simulink model "incre_encoder_new"  (R2020b)
settings: Solver=FixedStepDiscrete  StartTime=0.0  StopTime=0.15  RelTol=1e-3
undefined symbols (not defined in the file): DiscIntNeverNeededParam
libraries: simulink x13, hdlsllib x7
settings Model: DataTypeOverride=Off  Creator=ts  LastModifiedBy=ts
settings DataIOCC: LimitDataPoints=on  SaveOutput=off  SaveTime=off
settings OptimizationCC: BlockReduction=off  ConditionallyExecuteInputs=off  DefaultParameterBehavior=Inlined  LifeSpan=inf
settings DebuggingCC: AlgebraicLoopMsg=error  SingleTaskRateTransMsg=error  AllowSymbolicDim=off  StrictBusMsg=ErrorOnBusTreatedAsVector  SFUnexpectedBacktrackingDiag=warning  SFNoUnconditionalDefaultTransitionDiag=warning  SFExecutionAtInitializationDiag=none  ArithmeticOperatorsInVariantConditions=warning
settings HardwareCC: ProdBitPerPointer=32  ProdBitPerSizeT=32  ProdBitPerPtrDiffT=32  ProdLargestAtomicFloat=None  ProdIntDivRoundTo=Undefined  ProdEndianess=Unspecified  ProdWordSize=32  ProdHWDeviceType=ASIC/FPGA->ASIC/FPGA  ProdEqTarget=off
settings SFSimCC: SimUseLocalCustomCode=off  CustomCodeUndefinedFunction=UseInterfaceOnly
settings RTWCC: RTWUseLocalCustomCode=off
settings CodeAppCC: StateflowObjectComments=on
settings GRTTargetCC: TargetLangStandard=C89/C90 (ANSI)
settings ConfigComp: CovScope=ReferencedModels  CovMetricSettings=dw  CovSaveCumulativeToWorkspaceVar=on  CovSaveSingleToWorkspaceVar=on  CovExternalEMLEnable=off  CovSFcnEnable=off

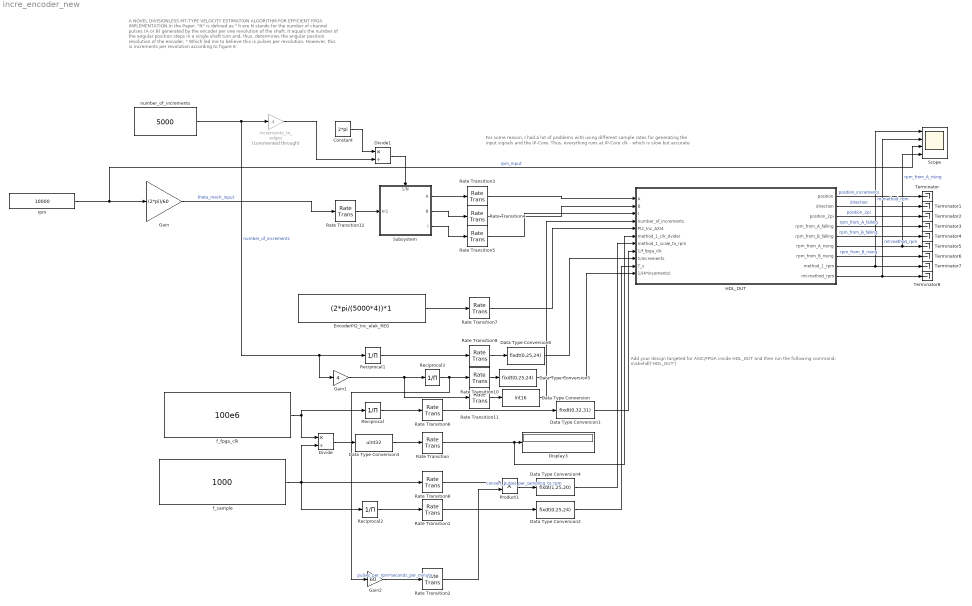
== system incre_encoder_new ==
  note: A NOVEL DIVISIONLESS MT-TYPE VELOCITY
      | ESTIMATION ALGORITHM FOR EFFICIENT
      | FPGA IMPLEMENTATION
      |
      | In the Paper, "N" is defined as " h ere N stands for the number of channel pulses (A or B) generated by the encoder per one revolution of the shaft. It
      | equals the number of the angular position steps in a single
      | shaft turn and, thus, determines the angular position resolution
      | of the encoder. "
      | Which led me to believe this is pulses per revolution. However, this is increments per revolution according to figure 6
  note: For some reason, I had a lot of problems with using different sample rates for generating the input signals and the IP-Core. Thus, everything runs at IP-Core clk - which is slow but accurate
  note: Add your design targeted for ASIC/FPGA inside HDL_DUT and then run the following command:
      | makehdl('HDL_DUT')
  Constant : Constant  Value=2*pi
  Data Type Conversion : DataTypeConversion  OutDataTypeStr=int16
  Data Type Conversion1 : DataTypeConversion  OutDataTypeStr=fixdt(0,32,31)
  Data Type Conversion2 : DataTypeConversion  OutMin=0  OutMax=0.01  OutDataTypeStr=fixdt(0,25,24)
  Data Type Conversion3 : DataTypeConversion  OutDataTypeStr=uint32
  Data Type Conversion4 : DataTypeConversion  OutDataTypeStr=fixdt(1,25,20)
  Data Type Conversion5 : DataTypeConversion  OutDataTypeStr=fixdt(0,25,24)
  Data Type Conversion6 : DataTypeConversion  OutDataTypeStr=fixdt(0,25,24)
  Display3 : Display
  Divide : Product  Inputs=*/
  Divide1 : Product  Inputs=*/
  EncoderPI2_Inc_elek_REG : Constant  Value=(2*pi/(5000*4))*1  OutDataTypeStr=fixdt(0,24,24)  SampleTime=-1
  Gain : Gain  Gain=(2*pi)/60
  Gain1 : Gain  Gain=4
  Gain2 : Gain  Gain=60
  HDL_DUT : Subsystem  TreatAsAtomicUnit=on
  Product1 : Product
  Rate Transition{,1..2,8,12} (5 alike) : RateTransition
  Rate Transition{3..7,9..11} (8 alike) : RateTransition  OutPortSampleTime=1/100e6
  Reciprocal{,1..3} (4 alike) : Product  Inputs=/
  Scope : Scope  NumInputPorts=4
  Subsystem : Subsystem
      settings: PortSchema="{\"entries\":[{\"content\":{\"sides\":[{\"content\":{\"connectorIds\":[\"In1\"]},\"type\":\"ConnectorPlacement.EquallySpacedRectSide\",\"uuid\":\"9e0d3c7a-ae59-4f05-b933-dde2182720d4\"},{\"content\":{\"connectorIds\":[\"Out1\",\"Out2\",\"Out3\"],\"side\":\"RIGHT\"},\"type\":\"ConnectorPlacement.EquallySpacedRectSide\",\"uuid\":\"061efe66-90e8-497d-a95d-e4bb14f2a7fd\"},{\"content\":{\"connectorIds\":[\"In2\"],\"side\":\"TOP\"},\"type\":\"ConnectorPlacement.EquallySpacedRectSide\",\"uuid\":\"3388cf49-edab-4489-bb14-c96d905dcdcb\"},{\"content\":{\"connectorIds\":[],\"side\":\"HIDDEN\"},\"type\":\"ConnectorPlacement.EquallySpacedRectSide\",\"uuid\":\"d7306302-0393-400a-9a2a-0d99055afcd2\"}]},\"type\":\"ConnectorPlacement.EquallySpacedConnector\",\"uuid\":\"eafc6ed9-e172-404f-862e-caf1c3fcd6e0\"}],\"packageUris\":[\"http://schema.mathworks.com/mf0/Connector/R2020b\"],\"version\":\"1.0\"}"
  Terminator{,1..8} (9 alike) : Terminator
  f_fpga_clk : Constant  Value=100e6
  f_sample : Constant  Value=1000
  increments_to_edges : Gain  Commented=through  Gain=4
  number_of_increments : Constant  Value=5000
  rpm : Constant  Value=10000
  wires:
  EncoderPI2_Inc_elek_REG/1 -> Rate Transition7/1
  Rate Transition3/1 -> HDL_DUT/1(A)
  Rate Transition4/1 -> HDL_DUT/2(B)
  Rate Transition5/1 -> HDL_DUT/3(I)
  Data Type Conversion/1 -> HDL_DUT/4(number_of_increments)
  Rate Transition7/1 -> HDL_DUT/5(PI2_Inc_AXI4)
  Product1/1 -> Data Type Conversion4/1  "convert_pulses_per_sampling_to_rpm"
  Rate Transition/1 -> HDL_DUT/6(method_1_clk_dvider), Display3/1
  Data Type Conversion3/1 -> Rate Transition/1
  f_fpga_clk/1 -> Reciprocal/1, Divide/1
  Divide/1 -> Data Type Conversion3/1
  Rate Transition8/1 -> Product1/1
  Reciprocal3/1 -> Gain2/1, Rate Transition10/1
  f_sample/1 -> Reciprocal2/1, Rate Transition8/1, Divide/2
  Rate Transition2/1 -> Product1/2
  Data Type Conversion4/1 -> HDL_DUT/7(method_1_scale_to_rpm)
  Gain/1 -> Rate Transition12/1  "theta_mech_input"
  number_of_increments/1 -> increments_to_edges/1, Gain1/1, Reciprocal1/1  "number_of_increments"
  Subsystem/1(A) -> Rate Transition3/1
  Subsystem/2(B) -> Rate Transition4/1
  Subsystem/3(I) -> Rate Transition5/1
  Reciprocal/1 -> Rate Transition6/1
  Reciprocal1/1 -> Rate Transition9/1
  Reciprocal2/1 -> Rate Transition1/1
  Rate Transition1/1 -> Data Type Conversion2/1
  HDL_DUT/1(position) -> Terminator/1  "position_increments"
  HDL_DUT/2(direction) -> Terminator1/1  "direction"
  HDL_DUT/3(position_2pi) -> Terminator2/1  "position_2pi"
  HDL_DUT/4(rpm_from_A_falling) -> Terminator3/1  "rpm_from_A_falling"
  HDL_DUT/5(rpm_from_B_falling) -> Terminator4/1  "rpm_from_B_falling"
  HDL_DUT/6(rpm_from_A_rising) -> Scope/4, Terminator5/1  "rpm_from_A_rising"
  HDL_DUT/7(rpm_from_B_rising) -> Terminator6/1  "rpm_from_B_rising"
  HDL_DUT/8(method_1_rpm) -> Scope/1, Terminator7/1  "m-method_rpm"
  HDL_DUT/9(mt-method_rpm) -> Scope/2, Terminator8/1  "mt-method_rpm"
  rpm/1 -> Scope/3, Gain/1  "rpm_input"
  Gain1/1 -> Rate Transition11/1, Reciprocal3/1
  Rate Transition9/1 -> Data Type Conversion6/1
  Rate Transition10/1 -> Data Type Conversion5/1
  Rate Transition11/1 -> Data Type Conversion/1
  Gain2/1 -> Rate Transition2/1  "pulses_per_rpm*seconds_per_minute"
  Rate Transition6/1 -> Data Type Conversion1/1
  Data Type Conversion1/1 -> HDL_DUT/8(1/f_fpga_clk)
  Data Type Conversion2/1 -> HDL_DUT/10(T_s)
  Data Type Conversion5/1 -> HDL_DUT/11(1/(4*incements))
  Data Type Conversion6/1 -> HDL_DUT/9(1/increments)
  Rate Transition12/1 -> Subsystem/1(In1)
  increments_to_edges/1 -> Divide1/2
  Divide1/1 -> Subsystem/2(1/N)
  Constant/1 -> Divide1/1

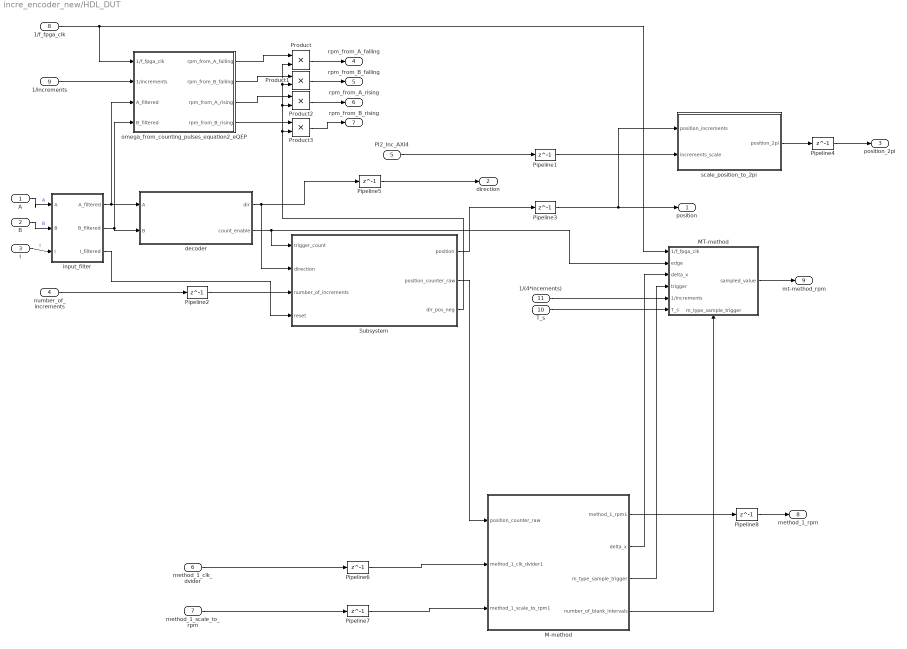
== system incre_encoder_new/HDL_DUT ==
  A : Inport
  B : Inport  Port=2
  I : Inport  Port=3
  number_of_increments : Inport  Port=4
  PI2_Inc_AXI4 : Inport  Port=5
  method_1_clk_dvider : Inport  Port=6
  method_1_scale_to_rpm : Inport  Port=7
  1/f_fpga_clk : Inport  Port=8
  1/increments : Inport  Port=9
  T_s : Inport  Port=10
  1/(4*incements) : Inport  Port=11
  M-method : Subsystem
  MT-method : Subsystem
      settings: PortSchema="{\"entries\":[{\"content\":{\"sides\":[{\"content\":{\"connectorIds\":[\"In1\",\"In2\",\"In3\",\"In4\",\"In5\",\"In6\"]},\"type\":\"ConnectorPlacement.EquallySpacedRectSide\",\"uuid\":\"ebb99f89-30f8-4ce6-b03f-8a2ff0950a3c\"},{\"content\":{\"connectorIds\":[\"Out1\"],\"side\":\"RIGHT\"},\"type\":\"ConnectorPlacement.EquallySpacedRectSide\",\"uuid\":\"75715ffe-4c0f-456c-8ce5-493fcfe41ee3\"},{\"content\":{\"connectorIds\":[],\"side\":\"TOP\"},\"type\":\"ConnectorPlacement.EquallySpacedRectSide\",\"uuid\":\"211c38e6-7e18-4a6c-98ce-7e5618ad5874\"},{\"content\":{\"connectorIds\":[\"In7\"],\"side\":\"BOTTOM\"},\"type\":\"ConnectorPlacement.EquallySpacedRectSide\",\"uuid\":\"87a6a744-1d19-4fed-b30a-33a6e99221e9\"},{\"content\":{\"connectorIds\":[],\"side\":\"HIDDEN\"},\"type\":\"ConnectorPlacement.EquallySpacedRectSide\",\"uuid\":\"5f32e9d6-05c7-4b0a-95ef-6efe95f3ff8d\"}]},\"type\":\"ConnectorPlacement.EquallySpacedConnector\",\"uuid\":\"473bacac-5052-4058-8fec-e1b83cc6224c\"}],\"packageUris\":[\"http://schema.mathworks.com/mf0/Connector/R2020b\"],\"version\":\"1.0\"}"
  Pipeline{1..8} (8 alike) : Delay  DelayLength=1
  Product{,1..3} (4 alike) : Product  OutDataTypeStr=fixdt(1,18,3)
  Subsystem : Subsystem
  decoder : Subsystem
  input_filter : Subsystem
  omega_from_counting_pulses_equation2_eQEP : Subsystem
  scale_position_to_2pi : Subsystem
  position : Outport  VectorParamsAs1DForOutWhenUnconnected=off
  direction : Outport  Port=2
  position_2pi : Outport  Port=3  VectorParamsAs1DForOutWhenUnconnected=off
  rpm_from_A_falling : Outport  Port=4
  rpm_from_B_falling : Outport  Port=5
  rpm_from_A_rising : Outport  Port=6
  rpm_from_B_rising : Outport  Port=7
  method_1_rpm : Outport  Port=8
  mt-method_rpm : Outport  Port=9
  wires:
  Pipeline3/1 -> position/1, scale_position_to_2pi/1(position_increments)
  input_filter/1(A_filtered) -> decoder/1(A), omega_from_counting_pulses_equation2_eQEP/3(A_filtered)
  decoder/1(dir) -> Pipeline5/1, Subsystem/2(direction)
  decoder/2(count_enable) -> Subsystem/1(trigger_count), MT-method/2(edge)
  input_filter/3(I_filtered) -> Subsystem/4(reset)
  Pipeline8/1 -> method_1_rpm/1
  Pipeline4/1 -> position_2pi/1
  Pipeline7/1 -> M-method/3(method_1_scale_to_rpm1)
  Pipeline1/1 -> scale_position_to_2pi/2(increments_scale)
  1/f_fpga_clk/1 -> omega_from_counting_pulses_equation2_eQEP/1(1/f_fpga_clk), MT-method/1(1/f_fpga_clk)
  B/1 -> input_filter/2(B)  "B"
  Pipeline5/1 -> direction/1
  PI2_Inc_AXI4/1 -> Pipeline1/1
  MT-method/1(sampled_value) -> mt-method_rpm/1
  scale_position_to_2pi/1(position_2pi) -> Pipeline4/1
  Subsystem/2(position_counter_raw) -> M-method/1(position_counter_raw)
  T_s/1 -> MT-method/6(T_s)
  A/1 -> input_filter/1(A)  "A"
  method_1_clk_dvider/1 -> Pipeline6/1
  input_filter/2(B_filtered) -> decoder/2(B), omega_from_counting_pulses_equation2_eQEP/4(B_filtered)
  Pipeline2/1 -> Subsystem/3(number_of_increments)
  method_1_scale_to_rpm/1 -> Pipeline7/1
  I/1 -> input_filter/3(I)  "I"
  Subsystem/1(position) -> Pipeline3/1
  Pipeline6/1 -> M-method/2(method_1_clk_dvider1)
  1/increments/1 -> omega_from_counting_pulses_equation2_eQEP/2(1/increments)
  number_of_increments/1 -> Pipeline2/1
  1/(4*incements)/1 -> MT-method/5(1/increments)
  M-method/4(number_of_blank_intervals) -> MT-method/7(m_type_sample_trigger)
  M-method/2(delta_x) -> MT-method/3(delta_x)
  M-method/3(m_type_sample_trigger) -> MT-method/4(trigger)
  M-method/1(method_1_rpm1) -> Pipeline8/1
  Product/1 -> rpm_from_A_falling/1
  Product1/1 -> rpm_from_B_falling/1
  Product2/1 -> rpm_from_A_rising/1
  Product3/1 -> rpm_from_B_rising/1
  Subsystem/3(dir_pos_neg) -> Product3/2, Product2/2, Product1/2, Product/2
  omega_from_counting_pulses_equation2_eQEP/4(rpm_from_B_rising) -> Product3/1
  omega_from_counting_pulses_equation2_eQEP/3(rpm_from_A_rising) -> Product2/1
  omega_from_counting_pulses_equation2_eQEP/2(rpm_from_B_falling) -> Product1/1
  omega_from_counting_pulses_equation2_eQEP/1(rpm_from_A_falling) -> Product/1

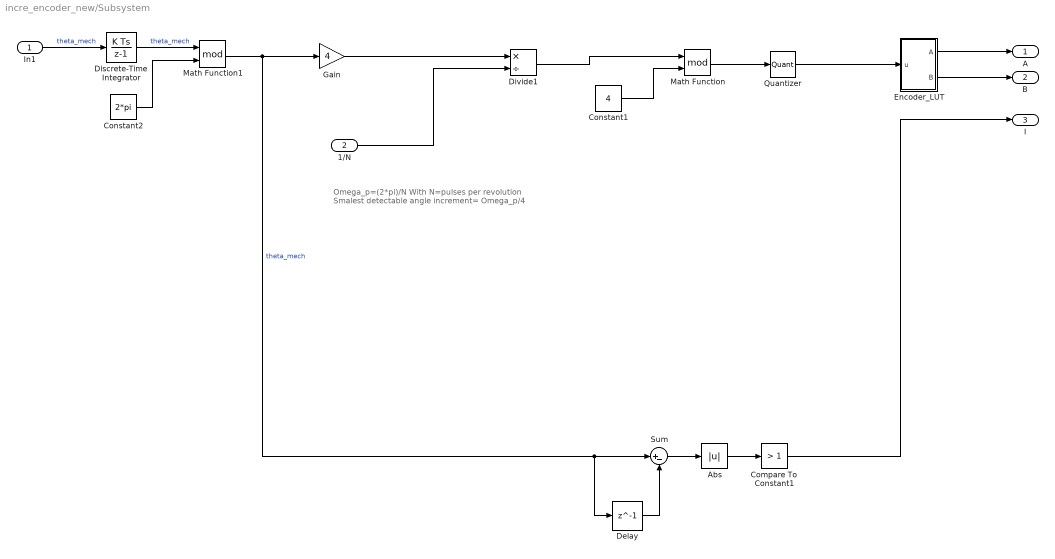
== system incre_encoder_new/Subsystem ==
  note: Omega_p=(2*pi)/N
      | With N=pulses per revolution
      | Smalest detectable angle increment= Omega_p/4
  In1 : Inport
  1/N : Inport  Port=2
  Abs : Abs
  Compare To Constant1 : simulink/Logic and Bit Operations/Compare To Constant  relop=>  const=1  OutDataTypeStr=boolean
  Constant1 : Constant  Value=4
  Constant2 : Constant  Value=2*pi  SampleTime=-1
  Delay : Delay  DelayLength=1
  Discrete-Time Integrator : DiscreteIntegrator  SampleTime=1/100000000  ICPrevOutput=DiscIntNeverNeededParam  ICPrevScaledInput=DiscIntNeverNeededParam
  Divide1 : Product  Inputs=*/
  Encoder_LUT : Subsystem
  Gain : Gain  Gain=4
  Math Function : Math  Operator=mod  SaturateOnIntegerOverflow=on
  Math Function1 : Math  Operator=mod  SaturateOnIntegerOverflow=on
  Quantizer : Quantizer  QuantizationInterval=1
  Sum : Sum  Inputs=|+-
  A : Outport
  B : Outport  Port=2
  I : Outport  Port=3
  wires:
  Gain/1 -> Divide1/1
  Divide1/1 -> Math Function/1
  Constant1/1 -> Math Function/2
  Math Function/1 -> Quantizer/1
  Quantizer/1 -> Encoder_LUT/1(u)
  Encoder_LUT/1(A) -> A/1
  Encoder_LUT/2(B) -> B/1
  Sum/1 -> Abs/1
  Delay/1 -> Sum/2
  Math Function1/1 -> Delay/1, Sum/1, Gain/1  "theta_mech"
  Abs/1 -> Compare To Constant1/1
  Compare To Constant1/1 -> I/1
  Discrete-Time Integrator/1 -> Math Function1/1  "theta_mech"
  Constant2/1 -> Math Function1/2
  In1/1 -> Discrete-Time Integrator/1  "theta_mech"
  1/N/1 -> Divide1/2

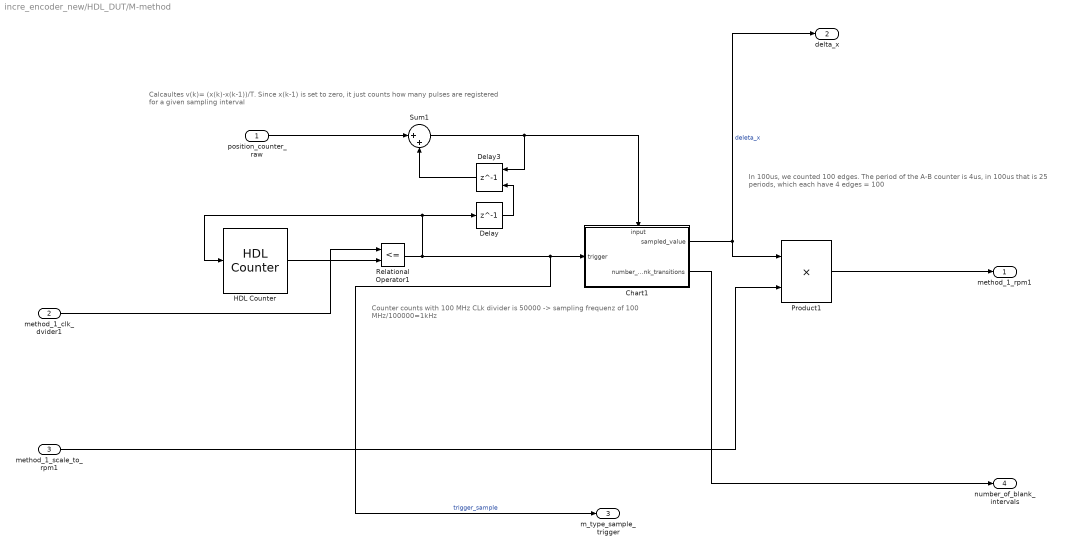
== system incre_encoder_new/HDL_DUT/M-method ==
  note: In 100us, we counted 100 edges.
      | The period of the A-B counter is 4us, in 100us that is 25 periods, which each have 4 edges = 100
  note: Counter counts with 100 MHz
      | CLk divider is 50000 -> sampling frequenz of 100 MHz/100000=1kHz
  note: Calcaultes v(k)= (x(k)-x(k-1))/T. Since x(k-1) is set to zero, it just counts how many pulses are registered for a given sampling interval
  position_counter_raw : Inport
  method_1_clk_dvider1 : Inport  Port=2
  method_1_scale_to_rpm1 : Inport  Port=3
  Chart1 : Stateflow chart  TreatAsAtomicUnit=on
      settings: PortSchema="{\"entries\":[{\"content\":{\"sides\":[{\"content\":{\"connectorIds\":[\"In2\"]},\"type\":\"ConnectorPlacement.EquallySpacedRectSide\",\"uuid\":\"939b8621-78f7-42aa-87b8-407a8b6a498a\"},{\"content\":{\"connectorIds\":[\"Out1\",\"Out2\"],\"side\":\"RIGHT\"},\"type\":\"ConnectorPlacement.EquallySpacedRectSide\",\"uuid\":\"3b067427-2d1d-4835-b293-703ef05eeccb\"},{\"content\":{\"connectorIds\":[\"In1\"],\"side\":\"TOP\"},\"type\":\"ConnectorPlacement.EquallySpacedRectSide\",\"uuid\":\"a3c90177-c936-46a5-9ed2-0ec0dd680635\"},{\"content\":{\"connectorIds\":[],\"side\":\"HIDDEN\"},\"type\":\"ConnectorPlacement.EquallySpacedRectSide\",\"uuid\":\"01f333f2-54e6-42b9-9b27-8dc26f013eb2\"}]},\"type\":\"ConnectorPlacement.EquallySpacedConnector\",\"uuid\":\"7e8a03bf-356f-48c3-b34e-0f0bd6eb938b\"}],\"packageUris\":[\"http://schema.mathworks.com/mf0/Connector/R2020b\"],\"version\":\"1.0\"}"
  Delay : Delay  DelayLength=1
  Delay3 : Delay  DelayLength=1  ExternalReset=Level
      settings: InputPortMap=u0,r5
  HDL Counter : hdlsllib/Sources/HDL Counter  CountType=Free running  CountInit=0  CountStep=1  CountMax=100  CountFromType=Initial value  CountFrom=0  CountResetPort=on  CountLoadPort=off  CountEnbPort=off  CountDirPort=off  CountDataType=Unsigned  CountWordLen=32  CountFracLen=0  CountSampTime=1
  Product1 : Product  OutDataTypeStr=fixdt(1,32,14)
  Relational Operator1 : RelationalOperator  Operator=<=  OutDataTypeStr=boolean  RndMeth=Simplest
  Sum1 : Sum  Inputs=|++  OutDataTypeStr=int32
  method_1_rpm1 : Outport
  delta_x : Outport  Port=2
  m_type_sample_trigger : Outport  Port=3
  number_of_blank_intervals : Outport  Port=4
  wires:
  method_1_scale_to_rpm1/1 -> Product1/2
  Chart1/1(sampled_value) -> Product1/1, delta_x/1  "deleta_x"
  Product1/1 -> method_1_rpm1/1
  position_counter_raw/1 -> Sum1/1
  Delay/1 -> Delay3/2
  Delay3/1 -> Sum1/2
  Sum1/1 -> Delay3/1, Chart1/1(input)
  method_1_clk_dvider1/1 -> Relational Operator1/1
  HDL Counter/1 -> Relational Operator1/2
  Relational Operator1/1 -> Delay/1, HDL Counter/1, m_type_sample_trigger/1, Chart1/2(trigger)  "trigger_sample"
  Chart1/2(number_of_blank_transitions) -> number_of_blank_intervals/1

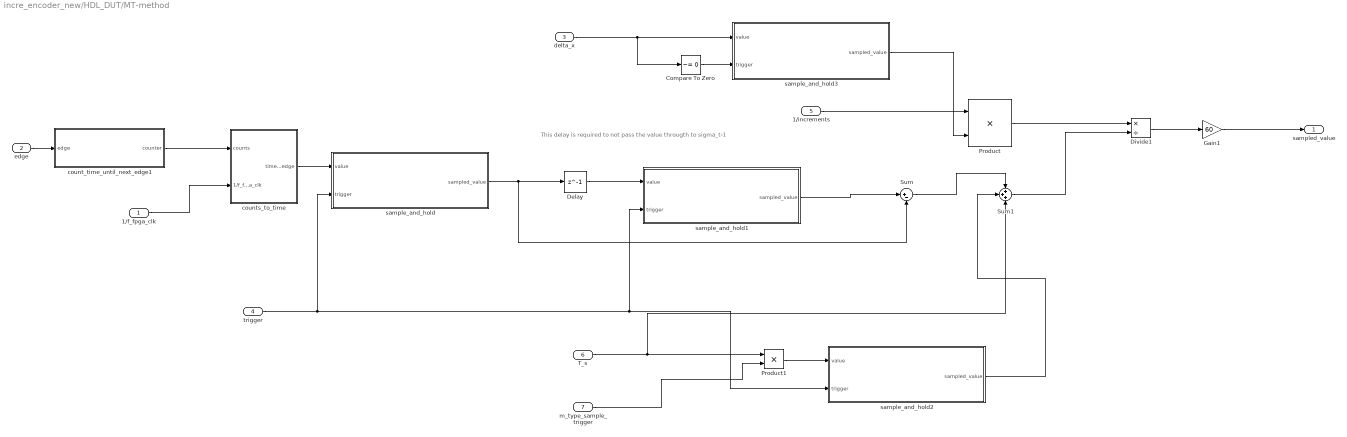
== system incre_encoder_new/HDL_DUT/MT-method ==
  note: This delay is required to not pass the value througth to sigma_t-1
  1/f_fpga_clk : Inport
  edge : Inport  Port=2
  delta_x : Inport  Port=3
  trigger : Inport  Port=4
  1/increments : Inport  Port=5
  T_s : Inport  Port=6
  m_type_sample_trigger : Inport  Port=7
  Compare To Zero : simulink/Logic and Bit Operations/Compare To Zero  relop=~=  OutDataTypeStr=boolean
  Delay : Delay  DelayLength=1
  Divide1 : Product  Inputs=*/  OutDataTypeStr=fixdt(1,18,4)
  Gain1 : Gain  Gain=60  OutDataTypeStr=fixdt(1,18,3)
  Product : Product
  Product1 : Product  OutDataTypeStr=Inherit: Same as first input
  Sum : Sum  Inputs=|+-
  Sum1 : Sum  Inputs=+++
  count_time_until_next_edge1 : Subsystem
  counts_to_time : Subsystem
  sample_and_hold : Subsystem
  sample_and_hold1 : Subsystem
  sample_and_hold2 : Subsystem
  sample_and_hold3 : Subsystem
  sampled_value : Outport
  wires:
  sample_and_hold/1(sampled_value) -> Delay/1, Sum/2
  sample_and_hold1/1(sampled_value) -> Sum/1
  count_time_until_next_edge1/1(counter) -> counts_to_time/1(counts)
  counts_to_time/1(time_since_last_edge) -> sample_and_hold/1(value)
  1/f_fpga_clk/1 -> counts_to_time/2(1/f_fpga_clk)
  delta_x/1 -> Compare To Zero/1, sample_and_hold3/1(value)
  Sum1/1 -> Divide1/2
  sample_and_hold2/1(sampled_value) -> Sum1/2
  Sum/1 -> Sum1/1
  Divide1/1 -> Gain1/1
  edge/1 -> count_time_until_next_edge1/1(edge)
  trigger/1 -> sample_and_hold/2(trigger), sample_and_hold2/2(trigger), sample_and_hold1/2(trigger)
  Delay/1 -> sample_and_hold1/1(value)
  1/increments/1 -> Product/1
  Product/1 -> Divide1/1
  T_s/1 -> Product1/1, Sum1/3
  m_type_sample_trigger/1 -> Product1/2
  Product1/1 -> sample_and_hold2/1(value)
  Compare To Zero/1 -> sample_and_hold3/2(trigger)
  Gain1/1 -> sampled_value/1
  sample_and_hold3/1(sampled_value) -> Product/2

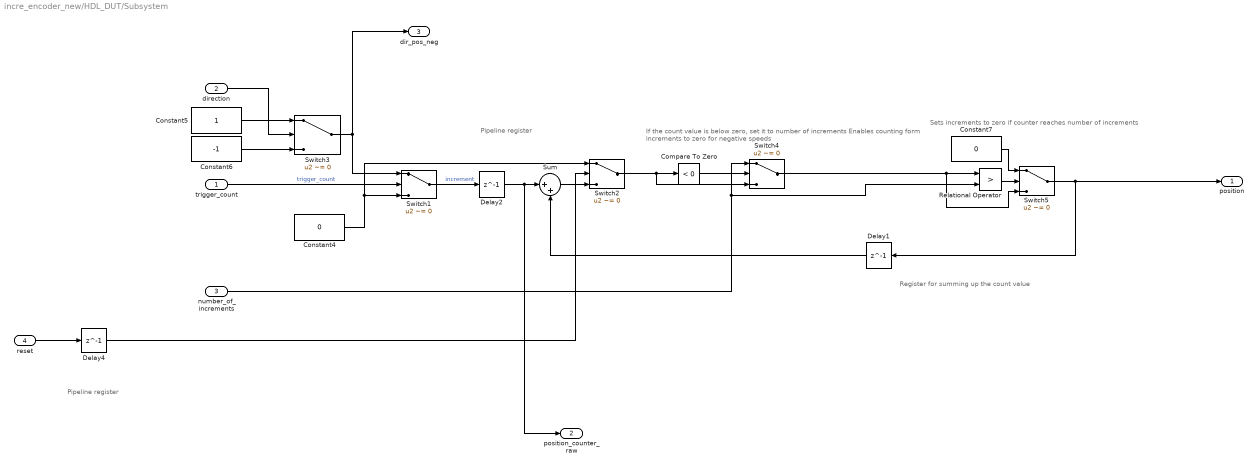
== system incre_encoder_new/HDL_DUT/Subsystem ==
  note: Pipeline register
  note: Register for summing up the count value
  note: Pipeline register
  note: If the count value is below zero, set it to number of increments
      | Enables counting form increments to zero for negative speeds
  note: Sets increments to zero if counter reaches number of increments
  trigger_count : Inport
  direction : Inport  Port=2
  number_of_increments : Inport  Port=3
  reset : Inport  Port=4
  Compare To Zero : simulink/Logic and Bit Operations/Compare To Zero  relop=<  OutDataTypeStr=boolean
  Constant4 : Constant  Value=0  OutDataTypeStr=Inherit: Inherit via back propagation  SampleTime=-1
  Constant5 : Constant  OutDataTypeStr=int16  SampleTime=-1
  Constant6 : Constant  Value=-1  OutDataTypeStr=int16  SampleTime=-1
  Constant7 : Constant  Value=0  OutDataTypeStr=int16  SampleTime=-1
  Delay1 : Delay  DelayLength=1
  Delay2 : Delay  DelayLength=1
  Delay4 : Delay  DelayLength=1
  Relational Operator : RelationalOperator  Operator=>  OutDataTypeStr=boolean  RndMeth=Nearest
  Sum : Sum  Inputs=|++  OutDataTypeStr=int16
  Switch{1..5} (5 alike) : Switch  Criteria=u2 ~= 0
  position : Outport
  position_counter_raw : Outport  Port=2
  dir_pos_neg : Outport  Port=3
  wires:
  Switch3/1 -> Switch1/1, dir_pos_neg/1
  Relational Operator/1 -> Switch5/2
  number_of_increments/1 -> Relational Operator/2, Switch4/1
  trigger_count/1 -> Switch1/2  "trigger_count"
  Constant7/1 -> Switch5/1
  direction/1 -> Switch3/2
  Switch2/1 -> Switch4/3, Compare To Zero/1
  Constant5/1 -> Switch3/1
  Switch5/1 -> position/1, Delay1/1
  Compare To Zero/1 -> Switch4/2
  Constant6/1 -> Switch3/3
  Switch1/1 -> Delay2/1  "increment"
  Delay1/1 -> Sum/2
  Switch4/1 -> Switch5/3, Relational Operator/1
  Constant4/1 -> Switch2/1, Switch1/3
  Sum/1 -> Switch2/3
  reset/1 -> Delay4/1
  Delay2/1 -> position_counter_raw/1, Sum/1
  Delay4/1 -> Switch2/2

== system incre_encoder_new/HDL_DUT/decoder ==
  A : Inport
  B : Inport  Port=2
  Bit Concat : hdlsllib/Logic and Bit Operations/Bit Concat  numInputs=2
  Chart : Stateflow chart  TreatAsAtomicUnit=on
      settings: PortSchema="{\"entries\":[{\"content\":{\"sides\":[{\"content\":{\"connectorIds\":[]},\"type\":\"ConnectorPlacement.EquallySpacedRectSide\",\"uuid\":\"daec34c6-1702-4005-aa49-10d4da34fe8f\"},{\"content\":{\"connectorIds\":[\"Out1\",\"Out2\"],\"side\":\"RIGHT\"},\"type\":\"ConnectorPlacement.EquallySpacedRectSide\",\"uuid\":\"001a9971-efab-40d0-ade0-c56900f25f3e\"},{\"content\":{\"connectorIds\":[\"In1\"],\"side\":\"TOP\"},\"type\":\"ConnectorPlacement.EquallySpacedRectSide\",\"uuid\":\"df9ef995-f205-435f-b234-17c3810a159e\"},{\"content\":{\"connectorIds\":[],\"side\":\"BOTTOM\"},\"type\":\"ConnectorPlacement.EquallySpacedRectSide\",\"uuid\":\"072d0b79-3392-4d8b-8dd8-d2187887a025\"},{\"content\":{\"connectorIds\":[],\"side\":\"HIDDEN\"},\"type\":\"ConnectorPlacement.EquallySpacedRectSide\",\"uuid\":\"c66a1be6-76cb-49b8-a915-e16581d132f1\"}]},\"type\":\"ConnectorPlacement.EquallySpacedConnector\",\"uuid\":\"6a8040ac-5c18-4913-8e6b-fe8fb202e8f4\"}],\"packageUris\":[\"http://schema.mathworks.com/mf0/Connector/R2020b\"],\"version\":\"1.0\"}"
  Detect Change : simulink/Logic and Bit Operations/Detect Change  vinit=0  OutDataTypeStr=boolean
  dir : Outport
  count_enable : Outport  Port=2
  wires:
  Chart/1(dir) -> dir/1  "dir"
  A/1 -> Bit Concat/2
  Bit Concat/1 -> Chart/1(state)  "state"
  Chart/2(count) -> Detect Change/1  "count_enable"
  B/1 -> Bit Concat/1
  Detect Change/1 -> count_enable/1  "trigger_count"

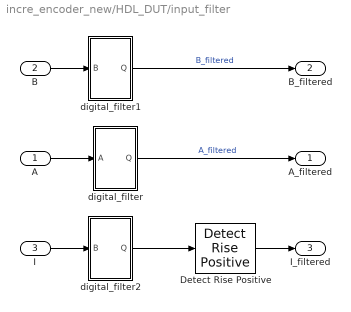
== system incre_encoder_new/HDL_DUT/input_filter ==
  A : Inport
  B : Inport  Port=2
  I : Inport  Port=3
  Detect Rise Positive : simulink/Logic and Bit Operations/Detect Rise Positive  vinit=0  OutDataTypeStr=boolean
  digital_filter : Subsystem
  digital_filter1 : Subsystem
  digital_filter2 : Subsystem
  A_filtered : Outport
  B_filtered : Outport  Port=2
  I_filtered : Outport  Port=3
  wires:
  digital_filter2/1(Q) -> Detect Rise Positive/1
  digital_filter1/1(Q) -> B_filtered/1  "B_filtered"
  B/1 -> digital_filter1/1(B)
  digital_filter/1(Q) -> A_filtered/1  "A_filtered"
  A/1 -> digital_filter/1(A)
  I/1 -> digital_filter2/1(B)
  Detect Rise Positive/1 -> I_filtered/1

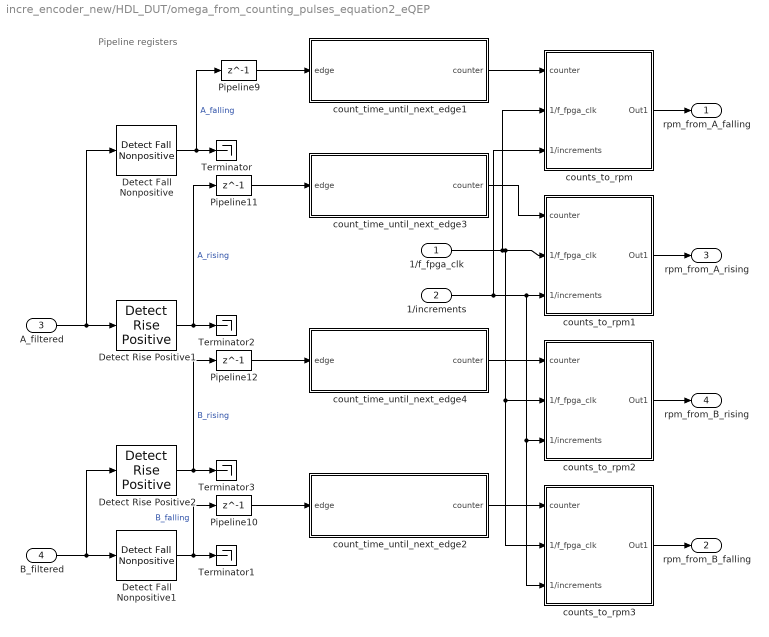
== system incre_encoder_new/HDL_DUT/omega_from_counting_pulses_equation2_eQEP ==
  note: Pipeline registers
  1/f_fpga_clk : Inport
  1/increments : Inport  Port=2
  A_filtered : Inport  Port=3
  B_filtered : Inport  Port=4
  Detect Fall Nonpositive : simulink/Logic and Bit Operations/Detect Fall Nonpositive  vinit=0  OutDataTypeStr=boolean
      settings: SourceProductBaseCode=SL
  Detect Fall Nonpositive1 : simulink/Logic and Bit Operations/Detect Fall Nonpositive  vinit=0  OutDataTypeStr=boolean
      settings: SourceProductBaseCode=SL
  Detect Rise Positive1 : simulink/Logic and Bit Operations/Detect Rise Positive  vinit=0  OutDataTypeStr=boolean
  Detect Rise Positive2 : simulink/Logic and Bit Operations/Detect Rise Positive  vinit=0  OutDataTypeStr=boolean
  Pipeline{9..12} (4 alike) : Delay  DelayLength=1
  Terminator{,1..3} (4 alike) : Terminator
  count_time_until_next_edge1 : Subsystem
  count_time_until_next_edge2 : Subsystem
  count_time_until_next_edge3 : Subsystem
  count_time_until_next_edge4 : Subsystem
  counts_to_rpm : Subsystem
  counts_to_rpm1 : Subsystem
  counts_to_rpm2 : Subsystem
  counts_to_rpm3 : Subsystem
  rpm_from_A_falling : Outport
  rpm_from_B_falling : Outport  Port=2
  rpm_from_A_rising : Outport  Port=3
  rpm_from_B_rising : Outport  Port=4
  wires:
  1/f_fpga_clk/1 -> counts_to_rpm1/2(1/f_fpga_clk), counts_to_rpm3/2(1/f_fpga_clk), counts_to_rpm2/2(1/f_fpga_clk), counts_to_rpm/2(1/f_fpga_clk)
  1/increments/1 -> counts_to_rpm1/3(1/increments), counts_to_rpm3/3(1/increments), counts_to_rpm2/3(1/increments), counts_to_rpm/3(1/increments)
  A_filtered/1 -> Detect Fall Nonpositive/1, Detect Rise Positive1/1
  Detect Fall Nonpositive/1 -> Pipeline9/1, Terminator/1  "A_falling"
  Detect Rise Positive2/1 -> Pipeline12/1, Terminator3/1  "B_rising"
  B_filtered/1 -> Detect Fall Nonpositive1/1, Detect Rise Positive2/1
  counts_to_rpm2/1(Out1) -> rpm_from_B_rising/1
  count_time_until_next_edge3/1(counter) -> counts_to_rpm1/1(counter)
  count_time_until_next_edge4/1(counter) -> counts_to_rpm2/1(counter)
  Detect Rise Positive1/1 -> Pipeline11/1, Terminator2/1  "A_rising"
  counts_to_rpm1/1(Out1) -> rpm_from_A_rising/1
  count_time_until_next_edge2/1(counter) -> counts_to_rpm3/1(counter)
  Pipeline9/1 -> count_time_until_next_edge1/1(edge)
  counts_to_rpm3/1(Out1) -> rpm_from_B_falling/1
  Pipeline10/1 -> count_time_until_next_edge2/1(edge)
  Pipeline11/1 -> count_time_until_next_edge3/1(edge)
  Pipeline12/1 -> count_time_until_next_edge4/1(edge)
  counts_to_rpm/1(Out1) -> rpm_from_A_falling/1
  count_time_until_next_edge1/1(counter) -> counts_to_rpm/1(counter)
  Detect Fall Nonpositive1/1 -> Pipeline10/1, Terminator1/1  "B_falling"

== system incre_encoder_new/HDL_DUT/scale_position_to_2pi ==
  note: Use position value after register to decrease critical path for the product
  position_increments : Inport
  increments_scale : Inport  Port=2
  Data Type Conversion : DataTypeConversion  OutDataTypeStr=fixdt(0,16,0)
  Product : Product  OutMin=0  OutMax=8  OutDataTypeStr=fixdt(0,32,27)
  position_2pi : Outport
  wires:
  Data Type Conversion/1 -> Product/1
  increments_scale/1 -> Product/2
  Product/1 -> position_2pi/1
  position_increments/1 -> Data Type Conversion/1

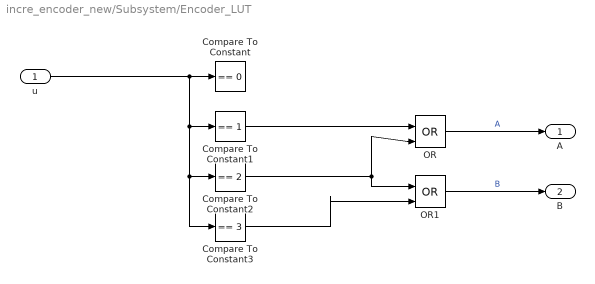
== system incre_encoder_new/Subsystem/Encoder_LUT ==
  u : Inport
  Compare To Constant : simulink/Logic and Bit Operations/Compare To Constant  relop===  const=0  OutDataTypeStr=boolean
  Compare To Constant1 : simulink/Logic and Bit Operations/Compare To Constant  relop===  const=1  OutDataTypeStr=boolean
  Compare To Constant2 : simulink/Logic and Bit Operations/Compare To Constant  relop===  const=2  OutDataTypeStr=boolean
  Compare To Constant3 : simulink/Logic and Bit Operations/Compare To Constant  relop===  const=3  OutDataTypeStr=boolean
  OR : Logic  Operator=OR  IconShape=distinctive  AllPortsSameDT=off  OutDataTypeStr=boolean
  OR1 : Logic  Operator=OR  IconShape=distinctive  AllPortsSameDT=off  OutDataTypeStr=boolean
  A : Outport
  B : Outport  Port=2
  wires:
  Compare To Constant3/1 -> OR1/2
  OR/1 -> A/1  "A"
  Compare To Constant1/1 -> OR/1
  Compare To Constant2/1 -> OR1/1, OR/2
  u/1 -> Compare To Constant3/1, Compare To Constant2/1, Compare To Constant1/1, Compare To Constant/1
  OR1/1 -> B/1  "B"

== system incre_encoder_new/HDL_DUT/MT-method/count_time_until_next_edge1 ==
  edge : Inport
  Delay : Delay  DelayLength=1
  HDL Counter : hdlsllib/Sources/HDL Counter  CountType=Free running  CountInit=0  CountStep=1  CountMax=25  CountFromType=Initial value  CountFrom=0  CountResetPort=on  CountLoadPort=off  CountEnbPort=off  CountDirPort=off  CountDataType=Unsigned  CountWordLen=32  CountFracLen=0  CountSampTime=1
  Switch : Switch  Criteria=u2 ~= 0
  counter : Outport
  wires:
  edge/1 -> Switch/2, HDL Counter/1
  Delay/1 -> Switch/3
  Switch/1 -> Delay/1, counter/1  "falling_counter"
  HDL Counter/1 -> Switch/1  "counts_since_edge"

== system incre_encoder_new/HDL_DUT/MT-method/counts_to_time ==
  note: Counts have to be multiplied by 1/f_fpga clock, e,g,. 10ns for 100MHz ip-core clk.
      | Than the inverse has to be multiplied by 1/increments of the encoder.
      | Result is scaled to rpm
  counts : Inport
  1/f_fpga_clk : Inport  Port=2
  Product : Product  OutDataTypeStr=fixdt(0,32,31)
  time_since_last_edge : Outport
  wires:
  counts/1 -> Product/1
  1/f_fpga_clk/1 -> Product/2
  Product/1 -> time_since_last_edge/1

== system incre_encoder_new/HDL_DUT/MT-method/sample_and_hold ==
  value : Inport
  trigger : Inport  Port=2
  Delay : Delay  DelayLength=1
  Switch : Switch  Criteria=u2 ~= 0
  sampled_value : Outport
  wires:
  trigger/1 -> Switch/2
  value/1 -> Switch/1
  Delay/1 -> Switch/3
  Switch/1 -> sampled_value/1, Delay/1  "falling_counter"

== system incre_encoder_new/HDL_DUT/MT-method/sample_and_hold1 ==
  value : Inport
  trigger : Inport  Port=2
  Delay : Delay  DelayLength=1
  Switch : Switch  Criteria=u2 ~= 0
  sampled_value : Outport
  wires:
  Switch/1 -> Delay/1, sampled_value/1  "falling_counter"
  Delay/1 -> Switch/3
  value/1 -> Switch/1
  trigger/1 -> Switch/2

== system incre_encoder_new/HDL_DUT/MT-method/sample_and_hold2 ==
  value : Inport
  trigger : Inport  Port=2
  Delay : Delay  DelayLength=1
  Switch : Switch  Criteria=u2 ~= 0
  sampled_value : Outport
  wires:
  trigger/1 -> Switch/2
  value/1 -> Switch/1
  Delay/1 -> Switch/3
  Switch/1 -> sampled_value/1, Delay/1  "falling_counter"

== system incre_encoder_new/HDL_DUT/MT-method/sample_and_hold3 ==
  value : Inport
  trigger : Inport  Port=2
  Delay : Delay  DelayLength=1
  Switch : Switch  Criteria=u2 ~= 0
  sampled_value : Outport
  wires:
  Switch/1 -> Delay/1, sampled_value/1  "falling_counter"
  Delay/1 -> Switch/3
  value/1 -> Switch/1
  trigger/1 -> Switch/2

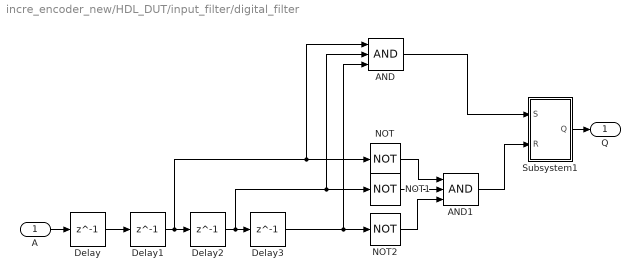
== system incre_encoder_new/HDL_DUT/input_filter/digital_filter ==
  A : Inport
  AND : Logic  Inputs=3  IconShape=distinctive  AllPortsSameDT=off  OutDataTypeStr=boolean
  AND1 : Logic  Inputs=3  IconShape=distinctive  AllPortsSameDT=off  OutDataTypeStr=boolean
  Delay{,1..3} (4 alike) : Delay  DelayLength=1
  NOT : Logic  Operator=NOT  IconShape=distinctive  AllPortsSameDT=off  OutDataTypeStr=boolean
  NOT1 : Logic  Operator=NOT  IconShape=distinctive  AllPortsSameDT=off  OutDataTypeStr=boolean
  NOT2 : Logic  Operator=NOT  IconShape=distinctive  AllPortsSameDT=off  OutDataTypeStr=boolean
  Subsystem1 : Subsystem
  Q : Outport
  wires:
  Delay/1 -> Delay1/1
  NOT2/1 -> AND1/3
  NOT1/1 -> AND1/2
  NOT/1 -> AND1/1
  Delay3/1 -> AND/3, NOT2/1
  Delay2/1 -> AND/2, NOT1/1, Delay3/1
  Delay1/1 -> AND/1, NOT/1, Delay2/1
  A/1 -> Delay/1
  Subsystem1/1(Q) -> Q/1
  AND1/1 -> Subsystem1/2(R)
  AND/1 -> Subsystem1/1(S)

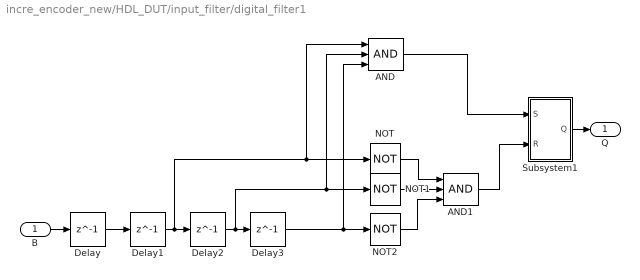
== system incre_encoder_new/HDL_DUT/input_filter/digital_filter1 ==
  B : Inport
  AND : Logic  Inputs=3  IconShape=distinctive  AllPortsSameDT=off  OutDataTypeStr=boolean
  AND1 : Logic  Inputs=3  IconShape=distinctive  AllPortsSameDT=off  OutDataTypeStr=boolean
  Delay{,1..3} (4 alike) : Delay  DelayLength=1
  NOT : Logic  Operator=NOT  IconShape=distinctive  AllPortsSameDT=off  OutDataTypeStr=boolean
  NOT1 : Logic  Operator=NOT  IconShape=distinctive  AllPortsSameDT=off  OutDataTypeStr=boolean
  NOT2 : Logic  Operator=NOT  IconShape=distinctive  AllPortsSameDT=off  OutDataTypeStr=boolean
  Subsystem1 : Subsystem
  Q : Outport
  wires:
  Subsystem1/1(Q) -> Q/1
  B/1 -> Delay/1
  Delay1/1 -> Delay2/1, NOT/1, AND/1
  Delay2/1 -> Delay3/1, NOT1/1, AND/2
  AND1/1 -> Subsystem1/2(R)
  Delay3/1 -> NOT2/1, AND/3
  NOT/1 -> AND1/1
  NOT1/1 -> AND1/2
  AND/1 -> Subsystem1/1(S)
  NOT2/1 -> AND1/3
  Delay/1 -> Delay1/1

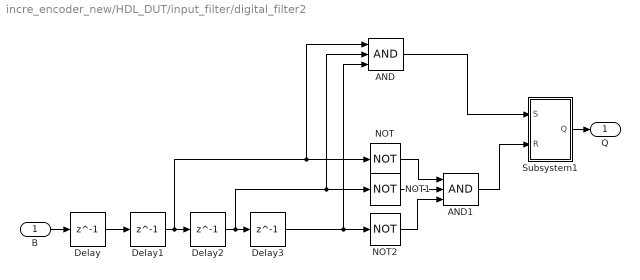
== system incre_encoder_new/HDL_DUT/input_filter/digital_filter2 ==
  B : Inport
  AND : Logic  Inputs=3  IconShape=distinctive  AllPortsSameDT=off  OutDataTypeStr=boolean
  AND1 : Logic  Inputs=3  IconShape=distinctive  AllPortsSameDT=off  OutDataTypeStr=boolean
  Delay{,1..3} (4 alike) : Delay  DelayLength=1
  NOT : Logic  Operator=NOT  IconShape=distinctive  AllPortsSameDT=off  OutDataTypeStr=boolean
  NOT1 : Logic  Operator=NOT  IconShape=distinctive  AllPortsSameDT=off  OutDataTypeStr=boolean
  NOT2 : Logic  Operator=NOT  IconShape=distinctive  AllPortsSameDT=off  OutDataTypeStr=boolean
  Subsystem1 : Subsystem
  Q : Outport
  wires:
  Delay/1 -> Delay1/1
  NOT2/1 -> AND1/3
  AND/1 -> Subsystem1/1(S)
  NOT1/1 -> AND1/2
  NOT/1 -> AND1/1
  Delay3/1 -> AND/3, NOT2/1
  AND1/1 -> Subsystem1/2(R)
  Delay2/1 -> AND/2, NOT1/1, Delay3/1
  Delay1/1 -> AND/1, NOT/1, Delay2/1
  B/1 -> Delay/1
  Subsystem1/1(Q) -> Q/1

== system incre_encoder_new/HDL_DUT/omega_from_counting_pulses_equation2_eQEP/count_time_until_next_edge1 ==
  edge : Inport
  Delay : Delay  DelayLength=1
  HDL Counter : hdlsllib/Sources/HDL Counter  CountType=Free running  CountInit=0  CountStep=1  CountMax=25  CountFromType=Initial value  CountFrom=0  CountResetPort=on  CountLoadPort=off  CountEnbPort=off  CountDirPort=off  CountDataType=Unsigned  CountWordLen=32  CountFracLen=0  CountSampTime=1
  Switch : Switch  Criteria=u2 ~= 0
  counter : Outport
  wires:
  edge/1 -> Switch/2, HDL Counter/1
  Delay/1 -> Switch/3
  Switch/1 -> Delay/1, counter/1  "falling_counter"
  HDL Counter/1 -> Switch/1  "counts_since_edge"

== system incre_encoder_new/HDL_DUT/omega_from_counting_pulses_equation2_eQEP/count_time_until_next_edge2 ==
  edge : Inport
  Delay : Delay  DelayLength=1
  HDL Counter : hdlsllib/Sources/HDL Counter  CountType=Free running  CountInit=0  CountStep=1  CountMax=25  CountFromType=Initial value  CountFrom=0  CountResetPort=on  CountLoadPort=off  CountEnbPort=off  CountDirPort=off  CountDataType=Unsigned  CountWordLen=32  CountFracLen=0  CountSampTime=1
  Switch : Switch  Criteria=u2 ~= 0
  counter : Outport
  wires:
  HDL Counter/1 -> Switch/1  "counts_since_edge"
  Switch/1 -> counter/1, Delay/1  "falling_counter"
  Delay/1 -> Switch/3
  edge/1 -> HDL Counter/1, Switch/2

== system incre_encoder_new/HDL_DUT/omega_from_counting_pulses_equation2_eQEP/count_time_until_next_edge3 ==
  edge : Inport
  Delay : Delay  DelayLength=1
  HDL Counter : hdlsllib/Sources/HDL Counter  CountType=Free running  CountInit=0  CountStep=1  CountMax=25  CountFromType=Initial value  CountFrom=0  CountResetPort=on  CountLoadPort=off  CountEnbPort=off  CountDirPort=off  CountDataType=Unsigned  CountWordLen=32  CountFracLen=0  CountSampTime=1
  Switch : Switch  Criteria=u2 ~= 0
  counter : Outport
  wires:
  edge/1 -> Switch/2, HDL Counter/1
  Delay/1 -> Switch/3
  Switch/1 -> Delay/1, counter/1  "falling_counter"
  HDL Counter/1 -> Switch/1  "counts_since_edge"

== system incre_encoder_new/HDL_DUT/omega_from_counting_pulses_equation2_eQEP/count_time_until_next_edge4 ==
  edge : Inport
  Delay : Delay  DelayLength=1
  HDL Counter : hdlsllib/Sources/HDL Counter  CountType=Free running  CountInit=0  CountStep=1  CountMax=25  CountFromType=Initial value  CountFrom=0  CountResetPort=on  CountLoadPort=off  CountEnbPort=off  CountDirPort=off  CountDataType=Unsigned  CountWordLen=32  CountFracLen=0  CountSampTime=1
  Switch : Switch  Criteria=u2 ~= 0
  counter : Outport
  wires:
  HDL Counter/1 -> Switch/1  "counts_since_edge"
  Switch/1 -> counter/1, Delay/1  "falling_counter"
  Delay/1 -> Switch/3
  edge/1 -> HDL Counter/1, Switch/2

== system incre_encoder_new/HDL_DUT/omega_from_counting_pulses_equation2_eQEP/counts_to_rpm ==
  note: Counts have to be multiplied by 1/f_fpga clock, e,g,. 10ns for 100MHz ip-core clk.
      | Than the inverse has to be multiplied by 1/increments of the encoder.
      | Result is scaled to rpm
  counter : Inport
  1/f_fpga_clk : Inport  Port=2
  1/increments : Inport  Port=3
  HDL Reciprocal : Reciprocal
  Product : Product  OutDataTypeStr=Inherit: Same as first input
  Product1 : Product  OutDataTypeStr=fixdt(0,18,10)
  to_rpms : Gain  Gain=60  OutDataTypeStr=fixdt(0,18,4)
  Out1 : Outport
  wires:
  Product1/1 -> to_rpms/1
  HDL Reciprocal/1 -> Product1/2
  Product/1 -> HDL Reciprocal/1
  counter/1 -> Product/2
  to_rpms/1 -> Out1/1
  1/f_fpga_clk/1 -> Product/1
  1/increments/1 -> Product1/1

== system incre_encoder_new/HDL_DUT/omega_from_counting_pulses_equation2_eQEP/counts_to_rpm1 ==
  note: Counts have to be multiplied by 1/f_fpga clock, e,g,. 10ns for 100MHz ip-core clk.
      | Than the inverse has to be multiplied by 1/increments of the encoder.
      | Result is scaled to rpm
  counter : Inport
  1/f_fpga_clk : Inport  Port=2
  1/increments : Inport  Port=3
  HDL Reciprocal : Reciprocal
  Product : Product  OutDataTypeStr=Inherit: Same as first input
  Product1 : Product  OutDataTypeStr=fixdt(0,18,10)
  to_rpms : Gain  Gain=60  OutDataTypeStr=fixdt(0,18,4)
  Out1 : Outport
  wires:
  1/increments/1 -> Product1/1
  1/f_fpga_clk/1 -> Product/1
  to_rpms/1 -> Out1/1
  counter/1 -> Product/2
  Product/1 -> HDL Reciprocal/1
  HDL Reciprocal/1 -> Product1/2
  Product1/1 -> to_rpms/1

== system incre_encoder_new/HDL_DUT/omega_from_counting_pulses_equation2_eQEP/counts_to_rpm2 ==
  note: Counts have to be multiplied by 1/f_fpga clock, e,g,. 10ns for 100MHz ip-core clk.
      | Than the inverse has to be multiplied by 1/increments of the encoder.
      | Result is scaled to rpm
  counter : Inport
  1/f_fpga_clk : Inport  Port=2
  1/increments : Inport  Port=3
  HDL Reciprocal : Reciprocal
  Product : Product  OutDataTypeStr=Inherit: Same as first input
  Product1 : Product  OutDataTypeStr=fixdt(0,18,10)
  to_rpms : Gain  Gain=60  OutDataTypeStr=fixdt(0,18,4)
  Out1 : Outport
  wires:
  Product1/1 -> to_rpms/1
  HDL Reciprocal/1 -> Product1/2
  Product/1 -> HDL Reciprocal/1
  counter/1 -> Product/2
  to_rpms/1 -> Out1/1
  1/f_fpga_clk/1 -> Product/1
  1/increments/1 -> Product1/1

== system incre_encoder_new/HDL_DUT/omega_from_counting_pulses_equation2_eQEP/counts_to_rpm3 ==
  note: Counts have to be multiplied by 1/f_fpga clock, e,g,. 10ns for 100MHz ip-core clk.
      | Than the inverse has to be multiplied by 1/increments of the encoder.
      | Result is scaled to rpm
  counter : Inport
  1/f_fpga_clk : Inport  Port=2
  1/increments : Inport  Port=3
  HDL Reciprocal : Reciprocal
  Product : Product  OutDataTypeStr=Inherit: Same as first input
  Product1 : Product  OutDataTypeStr=fixdt(0,18,10)
  to_rpms : Gain  Gain=60  OutDataTypeStr=fixdt(0,18,4)
  Out1 : Outport
  wires:
  1/increments/1 -> Product1/1
  1/f_fpga_clk/1 -> Product/1
  to_rpms/1 -> Out1/1
  counter/1 -> Product/2
  Product/1 -> HDL Reciprocal/1
  HDL Reciprocal/1 -> Product1/2
  Product1/1 -> to_rpms/1

== system incre_encoder_new/HDL_DUT/input_filter/digital_filter/Subsystem1 ==
  S : Inport
  R : Inport  Port=2
  AND : Logic  Operator=NOR  IconShape=distinctive  AllPortsSameDT=off  OutDataTypeStr=boolean
  AND1 : Logic  Operator=NOR  IconShape=distinctive  AllPortsSameDT=off  OutDataTypeStr=boolean
  Delay : Delay  DelayLength=1
  Q : Outport
  wires:
  S/1 -> AND1/2
  R/1 -> AND/1
  AND1/1 -> AND/2
  AND/1 -> Delay/1, Q/1
  Delay/1 -> AND1/1

== system incre_encoder_new/HDL_DUT/input_filter/digital_filter1/Subsystem1 ==
  S : Inport
  R : Inport  Port=2
  AND : Logic  Operator=NOR  IconShape=distinctive  AllPortsSameDT=off  OutDataTypeStr=boolean
  AND1 : Logic  Operator=NOR  IconShape=distinctive  AllPortsSameDT=off  OutDataTypeStr=boolean
  Delay : Delay  DelayLength=1
  Delay1 : Delay  DelayLength=1
  Q : Outport
  wires:
  Delay1/1 -> AND1/1
  Delay/1 -> AND/2
  S/1 -> AND/1
  R/1 -> AND1/2
  AND1/1 -> Delay/1
  AND/1 -> Delay1/1, Q/1

== system incre_encoder_new/HDL_DUT/input_filter/digital_filter2/Subsystem1 ==
  S : Inport
  R : Inport  Port=2
  AND : Logic  Operator=NOR  IconShape=distinctive  AllPortsSameDT=off  OutDataTypeStr=boolean
  AND1 : Logic  Operator=NOR  IconShape=distinctive  AllPortsSameDT=off  OutDataTypeStr=boolean
  Delay : Delay  DelayLength=1
  Delay1 : Delay  DelayLength=1
  Q : Outport
  wires:
  AND/1 -> Q/1, Delay1/1
  AND1/1 -> Delay/1
  R/1 -> AND1/2
  S/1 -> AND/1
  Delay/1 -> AND/2
  Delay1/1 -> AND1/1

== stateflow chart incre_encoder_new/HDL_DUT/M-method/Chart1 ==
  settings: stateMachineType=MEALY_MACHINE  executeAtInitialization=1
  state running
  state sample_value
  state blank_interval
  (default) -> running : {number_of_blank_transitions=int32(0)}
  blank_interval -> running
  sample_value -> running [order 1] : [sampled_value ~= int32(0)]{number_of_blank_transitions=int32(0)}
  running -> sample_value : [trigger==true]{sampled_value=input;}
  sample_value -> blank_interval [order 2] : [sampled_value==int32(0)]{number_of_blank_transitions=number_of_blank_transitions+int32(1)}
  data: input input; trigger input; sampled_value output; number_of_blank_transitions output

== stateflow chart incre_encoder_new/HDL_DUT/decoder/Chart ==
  settings: updateMethod=DISCRETE  stateMachineType=MEALY_MACHINE  executeAtInitialization=1
  state init
  state S00_0
  state S01_1
  state S10_2
  state S11_3
  init -> S10_2 [order 2] : [state==fi(2,0,2,0,hdlfimath)]
  (default) -> init : {count=false}
  init -> S00_0 [order 1] : [state==fi(0,0,2,0,hdlfimath)]
  init -> S01_1 [order 4] : [state==fi(1,0,2,0,hdlfimath)]
  init -> S11_3 [order 3] : [state==fi(3,0,2,0,hdlfimath)]
  S00_0 -> S01_1 [order 2] : [state==fi(1,0,2,0,hdlfimath)] {dir=false;count = ~count;}
  S10_2 -> S00_0 [order 2] : [state==fi(0,0,2,0,hdlfimath)] {dir=false;count = ~count;}
  S01_1 -> S00_0 [order 1] : [state==fi(0,0,2,0,hdlfimath)]{dir=true;count = ~count;}
  S00_0 -> S10_2 [order 1] : [state==fi(2,0,2,0,hdlfimath)] {dir=true;count = ~count;}
  S10_2 -> S11_3 [order 1] : [state==fi(3,0,2,0,hdlfimath)]{dir=true;count = ~count;}
  S11_3 -> S10_2 [order 2] : [state==fi(2,0,2,0,hdlfimath)] {dir=false;count = ~count;}
  S01_1 -> S11_3 [order 2] : [state==fi(3,0,2,0,hdlfimath)] {dir=false;count = ~count;}
  S11_3 -> S01_1 [order 1] : [state==fi(1,0,2,0,hdlfimath)]{dir=true;count = ~count;}
  data: state input; dir output; count output
